simulink model "ASM_Traffic_V2X_Complete_Model_2"  (R2019a)
settings: Solver=ode1  StartTime=SIM.tstart.v  StopTime=Inf  FixedStep=SIM.StepSize.v  RelTol=1e-3
PostLoadFcn:
  | if any(exist('dsrtsu_mdlpostloadfcn', 'file') ~= 0), dsrtsu_mdlpostloadfcn('Execute', bdroot); end
  | try, asm_mdl_postloadfcn(bdroot, 'UpdateModel', 2200); catch, disp(lasterr); end,
undefined symbols (not defined in the file): _SensorPnts_1, _SensorPnts_13, _SensorPnts_17, _SensorPnts_21, _SensorPnts_25, _SensorPnts_29, _SensorPnts_33, _SensorPnts_37, _SensorPnts_41, _SensorPnts_45, _SensorPnts_49, _SensorPnts_5, _SensorPnts_53, _SensorPnts_57, _SensorPnts_9, _to_, CPT, G5A, ITS, MDL, rad, s_to_rpm, SIM
libraries: simulink x169, ASM_VehicleDynamics_lib x126, ASM_Traffic_lib x83, ASM_Utils_lib x49, mdbs x45, ASM_Environment_lib x17, dspindex x12, dsaV2xLibraryAux x10, dsmpblib x6, dsaV2xAsn1Library x4, dsaV2xLibrary x4, ASM_BrakeHydraulics_lib x4
(part 34 of 36)

== system ASM_Traffic_V2X_Complete_Model_2/MDL/Environment/Traffic/Sensors/Object_Sensor_3D/RadarEffects/Sensor1/RadarEffectsOutput/ResetPulse ==
  Enable[0|1] : Inport
  SensorActive[0|1] : Inport  Port=2
  Compare To Constant : simulink/Logic and Bit Operations/Compare To Constant  relop===  const=1  OutDataTypeStr=boolean
  Compare To Constant1 : simulink/Logic and Bit Operations/Compare To Constant  relop===  const=0  OutDataTypeStr=boolean
  Logical Operator1 : Logic  AllPortsSameDT=off  OutDataTypeStr=boolean
  Logical Operator2 : Logic  Operator=NAND  AllPortsSameDT=off  OutDataTypeStr=boolean
  Memory1 : Memory
  ResetPulse[0|1] : Outport
  wires:
  Memory1/1 -> Compare To Constant1/1
  Logical Operator2/1 -> Compare To Constant/1, Memory1/1
  SensorActive[0|1]/1 -> Logical Operator2/1
  Logical Operator1/1 -> ResetPulse[0|1]/1
  Compare To Constant/1 -> Logical Operator1/1
  Compare To Constant1/1 -> Logical Operator1/2
  Enable[0|1]/1 -> Logical Operator2/2

== system ASM_Traffic_V2X_Complete_Model_2/MDL/Environment/Traffic/Sensors/Object_Sensor_3D/RadarEffects/Sensor1/RadarEffectsOutput/SignalBus ==
  RadarEffect_Signals_In[] : Inport
  Bus Creator : BusCreator  Inputs=5
  Bus Selector1 : BusSelector  OutputSignals=ID[],Object_ID[],Dist_CoorSys_S[m],Angle_Hor_CoorSys_S[deg],Pos_ObjectPoint_CoorSys_E[x;y;z][m]
  RadarEffect_Signals_Out[] : Outport
  wires:
  RadarEffect_Signals_In[]/1 -> Bus Selector1/1
  Bus Creator/1 -> RadarEffect_Signals_Out[]/1
  Bus Selector1/4 -> Bus Creator/4  "<Angle_Hor_CoorSys_S[deg]>"
  Bus Selector1/5 -> Bus Creator/5  "<Pos_ObjectPoint_CoorSys_E[x;y;z][m]>"
  Bus Selector1/2 -> Bus Creator/2  "<Object_ID[]>"
  Bus Selector1/3 -> Bus Creator/3  "<Dist_CoorSys_S[m]>"
  Bus Selector1/1 -> Bus Creator/1  "<ID[]>"

== system ASM_Traffic_V2X_Complete_Model_2/MDL/Environment/Traffic/Sensors/Object_Sensor_3D/RadarEffects/Sensor2/RadarEffectsOutput/HoldSignals ==
  ResetPulse[0|1] : Inport
  RadarEffect_Signals_In[] : Inport  Port=2
  Enable : EnablePort
  Bus Selector1 : BusSelector  OutputSignals=ID[],Dist_CoorSys_S[m],v_CoorSys_S[m|s],Angle_Hor_CoorSys_S[deg],Angle_Ver_CoorSys_S[deg],RCS[dBm2],Object_ID[],Object_Type[],Pos_ObjectPoint_CoorSys_E[x;y;z][m],Pos_ObjectPoint_CoorSys_S[x;y;z][m]
  RADAR_SIGNALS_RESET_2 : ASM_Traffic_lib/Sensors/RadarEffects/RADAR_SIGNALS_RESET  ASMProperties=struct('Name','RADAR_SIGNALS_RESET','Version','1.0','Library','ASM_Traffic_lib')  ASMInstanceName=radar_signals_reset  ASMInstanceID=1
  RadarEffect_Signals_Out[] : Outport
  wires:
  ResetPulse[0|1]/1 -> RADAR_SIGNALS_RESET_2/1
  Bus Selector1/8 -> RADAR_SIGNALS_RESET_2/9  "<Object_Type[]>"
  Bus Selector1/3 -> RADAR_SIGNALS_RESET_2/4  "<v_CoorSys_S[m|s]>"
  Bus Selector1/7 -> RADAR_SIGNALS_RESET_2/8  "<Object_ID[]>"
  RadarEffect_Signals_In[]/1 -> Bus Selector1/1
  Bus Selector1/6 -> RADAR_SIGNALS_RESET_2/7  "<RCS[dBm2]>"
  Bus Selector1/5 -> RADAR_SIGNALS_RESET_2/6  "<Angle_Ver_CoorSys_S[deg]>"
  Bus Selector1/4 -> RADAR_SIGNALS_RESET_2/5  "<Angle_Hor_CoorSys_S[deg]>"
  Bus Selector1/2 -> RADAR_SIGNALS_RESET_2/3  "<Dist_CoorSys_S[m]>"
  Bus Selector1/10 -> RADAR_SIGNALS_RESET_2/11  "<Pos_ObjectPoint_CoorSys_S[x;y;z][m]>"
  Bus Selector1/1 -> RADAR_SIGNALS_RESET_2/2  "<ID[]>"
  Bus Selector1/9 -> RADAR_SIGNALS_RESET_2/10  "<Pos_ObjectPoint_CoorSys_E[x;y;z][m]>"
  RADAR_SIGNALS_RESET_2/1 -> RadarEffect_Signals_Out[]/1

== system ASM_Traffic_V2X_Complete_Model_2/MDL/Environment/Traffic/Sensors/Object_Sensor_3D/RadarEffects/Sensor2/RadarEffectsOutput/ResetPulse ==
  Enable[0|1] : Inport
  SensorActive[0|1] : Inport  Port=2
  Compare To Constant : simulink/Logic and Bit Operations/Compare To Constant  relop===  const=1  OutDataTypeStr=boolean
  Compare To Constant1 : simulink/Logic and Bit Operations/Compare To Constant  relop===  const=0  OutDataTypeStr=boolean
  Logical Operator1 : Logic  AllPortsSameDT=off  OutDataTypeStr=boolean
  Logical Operator2 : Logic  Operator=NAND  AllPortsSameDT=off  OutDataTypeStr=boolean
  Memory1 : Memory
  ResetPulse[0|1] : Outport
  wires:
  Memory1/1 -> Compare To Constant1/1
  Logical Operator2/1 -> Compare To Constant/1, Memory1/1
  SensorActive[0|1]/1 -> Logical Operator2/1
  Logical Operator1/1 -> ResetPulse[0|1]/1
  Compare To Constant/1 -> Logical Operator1/1
  Compare To Constant1/1 -> Logical Operator1/2
  Enable[0|1]/1 -> Logical Operator2/2

== system ASM_Traffic_V2X_Complete_Model_2/MDL/Environment/Traffic/Sensors/Object_Sensor_3D/RadarEffects/Sensor2/RadarEffectsOutput/SignalBus ==
  RadarEffect_Signals_In[] : Inport
  Bus Creator : BusCreator  Inputs=5
  Bus Selector1 : BusSelector  OutputSignals=ID[],Object_ID[],Dist_CoorSys_S[m],Angle_Hor_CoorSys_S[deg],Pos_ObjectPoint_CoorSys_E[x;y;z][m]
  RadarEffect_Signals_Out[] : Outport
  wires:
  RadarEffect_Signals_In[]/1 -> Bus Selector1/1
  Bus Creator/1 -> RadarEffect_Signals_Out[]/1
  Bus Selector1/4 -> Bus Creator/4  "<Angle_Hor_CoorSys_S[deg]>"
  Bus Selector1/5 -> Bus Creator/5  "<Pos_ObjectPoint_CoorSys_E[x;y;z][m]>"
  Bus Selector1/2 -> Bus Creator/2  "<Object_ID[]>"
  Bus Selector1/3 -> Bus Creator/3  "<Dist_CoorSys_S[m]>"
  Bus Selector1/1 -> Bus Creator/1  "<ID[]>"

== system ASM_Traffic_V2X_Complete_Model_2/MDL/Environment/Traffic/Sensors/Object_Sensor_3D/RadarEffects/Sensor3/RadarEffectsOutput/HoldSignals ==
  ResetPulse[0|1] : Inport
  RadarEffect_Signals_In[] : Inport  Port=2
  Enable : EnablePort
  Bus Selector1 : BusSelector  OutputSignals=ID[],Dist_CoorSys_S[m],v_CoorSys_S[m|s],Angle_Hor_CoorSys_S[deg],Angle_Ver_CoorSys_S[deg],RCS[dBm2],Object_ID[],Object_Type[],Pos_ObjectPoint_CoorSys_E[x;y;z][m],Pos_ObjectPoint_CoorSys_S[x;y;z][m]
  RADAR_SIGNALS_RESET_3 : ASM_Traffic_lib/Sensors/RadarEffects/RADAR_SIGNALS_RESET  ASMProperties=struct('Name','RADAR_SIGNALS_RESET','Version','1.0','Library','ASM_Traffic_lib')  ASMInstanceName=radar_signals_reset  ASMInstanceID=1
  RadarEffect_Signals_Out[] : Outport
  wires:
  RADAR_SIGNALS_RESET_3/1 -> RadarEffect_Signals_Out[]/1
  Bus Selector1/9 -> RADAR_SIGNALS_RESET_3/10  "<Pos_ObjectPoint_CoorSys_E[x;y;z][m]>"
  Bus Selector1/5 -> RADAR_SIGNALS_RESET_3/6  "<Angle_Ver_CoorSys_S[deg]>"
  Bus Selector1/4 -> RADAR_SIGNALS_RESET_3/5  "<Angle_Hor_CoorSys_S[deg]>"
  Bus Selector1/1 -> RADAR_SIGNALS_RESET_3/2  "<ID[]>"
  ResetPulse[0|1]/1 -> RADAR_SIGNALS_RESET_3/1
  Bus Selector1/6 -> RADAR_SIGNALS_RESET_3/7  "<RCS[dBm2]>"
  Bus Selector1/7 -> RADAR_SIGNALS_RESET_3/8  "<Object_ID[]>"
  Bus Selector1/3 -> RADAR_SIGNALS_RESET_3/4  "<v_CoorSys_S[m|s]>"
  RadarEffect_Signals_In[]/1 -> Bus Selector1/1
  Bus Selector1/10 -> RADAR_SIGNALS_RESET_3/11  "<Pos_ObjectPoint_CoorSys_S[x;y;z][m]>"
  Bus Selector1/8 -> RADAR_SIGNALS_RESET_3/9  "<Object_Type[]>"
  Bus Selector1/2 -> RADAR_SIGNALS_RESET_3/3  "<Dist_CoorSys_S[m]>"

== system ASM_Traffic_V2X_Complete_Model_2/MDL/Environment/Traffic/Sensors/Object_Sensor_3D/RadarEffects/Sensor3/RadarEffectsOutput/ResetPulse ==
  Enable[0|1] : Inport
  SensorActive[0|1] : Inport  Port=2
  Compare To Constant : simulink/Logic and Bit Operations/Compare To Constant  relop===  const=1  OutDataTypeStr=boolean
  Compare To Constant1 : simulink/Logic and Bit Operations/Compare To Constant  relop===  const=0  OutDataTypeStr=boolean
  Logical Operator1 : Logic  AllPortsSameDT=off  OutDataTypeStr=boolean
  Logical Operator2 : Logic  Operator=NAND  AllPortsSameDT=off  OutDataTypeStr=boolean
  Memory1 : Memory
  ResetPulse[0|1] : Outport
  wires:
  Memory1/1 -> Compare To Constant1/1
  Logical Operator2/1 -> Compare To Constant/1, Memory1/1
  SensorActive[0|1]/1 -> Logical Operator2/1
  Logical Operator1/1 -> ResetPulse[0|1]/1
  Compare To Constant/1 -> Logical Operator1/1
  Compare To Constant1/1 -> Logical Operator1/2
  Enable[0|1]/1 -> Logical Operator2/2

== system ASM_Traffic_V2X_Complete_Model_2/MDL/Environment/Traffic/Sensors/Object_Sensor_3D/RadarEffects/Sensor3/RadarEffectsOutput/SignalBus ==
  RadarEffect_Signals_In[] : Inport
  Bus Creator : BusCreator  Inputs=5
  Bus Selector1 : BusSelector  OutputSignals=ID[],Object_ID[],Dist_CoorSys_S[m],Angle_Hor_CoorSys_S[deg],Pos_ObjectPoint_CoorSys_E[x;y;z][m]
  RadarEffect_Signals_Out[] : Outport
  wires:
  RadarEffect_Signals_In[]/1 -> Bus Selector1/1
  Bus Creator/1 -> RadarEffect_Signals_Out[]/1
  Bus Selector1/4 -> Bus Creator/4  "<Angle_Hor_CoorSys_S[deg]>"
  Bus Selector1/5 -> Bus Creator/5  "<Pos_ObjectPoint_CoorSys_E[x;y;z][m]>"
  Bus Selector1/2 -> Bus Creator/2  "<Object_ID[]>"
  Bus Selector1/3 -> Bus Creator/3  "<Dist_CoorSys_S[m]>"
  Bus Selector1/1 -> Bus Creator/1  "<ID[]>"

== system ASM_Traffic_V2X_Complete_Model_2/MDLUserInterface/MotionDeskInterface/MOTION_DESK_INTERFACE/Traffic_Animation/Sensors_Animation/Sensor_Points/Object_Sensor_2D_Points/Calc_Object_Sensor_2D_Points/Sensor_Points ==
  Transform_In : Inport
  Angle_Hor_Rel[deg] : Inport  Port=2
  Distance[m] : Inport  Port=3
  Num_SensorRays_Used[] : Inport  Port=4
  Add : Sum
  CheckUnusedPoints : RelationalOperator  Operator=<  OutDataTypeStr=boolean  RndMeth=Nearest
  Concatenate : Concatenate  NumInputs=4  Mode=Multidimensional array
  Constant1 : Constant  Value=0.99999
  Cos : Trigonometry  Operator=cos
  Deg2Rad : Gain  Gain=pi/180
  Demux : Demux
  Demux1 : Demux
  Demux2 : Demux
  DownAway : Constant  Value=-999999
  ForIterator_Current : Subsystem  TreatAsAtomicUnit=on
  Product{,1..6} (7 alike) : Product
  Reshape : Reshape  OutputDimensionality=Row vector (2-D)
  Reshape1 : Reshape  OutputDimensionality=Row vector (2-D)
  Reshape2 : Reshape  OutputDimensionality=Row vector (2-D)
  Row0 : Selector  NumberOfDimensions=2  IndexMode=Zero-based  InputPortWidth=3  IndexOptions=Index vector (dialog),Index vector (dialog)  Indices=0,-1  OutputSizes=1,1
  Row1 : Selector  NumberOfDimensions=2  IndexMode=Zero-based  InputPortWidth=3  IndexOptions=Index vector (dialog),Index vector (dialog)  Indices=1,-1  OutputSizes=1,1
  Row2 : Selector  NumberOfDimensions=2  IndexMode=Zero-based  InputPortWidth=3  IndexOptions=Index vector (dialog),Index vector (dialog)  Indices=2,-1  OutputSizes=1,1
  Sin : Trigonometry
  Term : Terminator
  Term1 : Terminator
  Term2 : Terminator
  X : Sum  Inputs=+++
  Y : Sum  Inputs=+++
  Z : Sum  Inputs=+++
  dim_animation_point[] : Constant  Value=60
  init_animation_point[] : Constant  Value=zeros(1,60)  VectorParams1D=off
  x1 : Product
  y1 : Product
  y2 : Product
  y3 : Product
  Translate[x;y;z][m] : Outport
  wires:
  CheckUnusedPoints/1 -> Product/1
  Constant1/1 -> CheckUnusedPoints/2
  Product/1 -> Add/1
  DownAway/1 -> Product/2
  Add/1 -> Concatenate/3
  Reshape2/1 -> Add/2
  ForIterator_Current/3(flag_point_used[0|1]) -> CheckUnusedPoints/1, y3/1, y2/2
  Z/1 -> Reshape2/1
  Demux2/4 -> Z/3
  Product5/1 -> Z/2
  Product6/1 -> Z/1
  Demux2/3 -> Term2/1
  Demux2/2 -> Product5/1
  Demux2/1 -> Product6/1
  Row2/1 -> Demux2/1
  Y/1 -> Reshape1/1
  X/1 -> Reshape/1
  Concatenate/1 -> Translate[x;y;z][m]/1
  Demux1/4 -> Y/3
  Product3/1 -> Y/2
  Product4/1 -> Y/1
  Demux1/3 -> Term1/1
  Demux1/2 -> Product3/1
  Demux1/1 -> Product4/1
  Row1/1 -> Demux1/1
  Demux/4 -> X/3
  Product1/1 -> X/2
  Product2/1 -> X/1
  Demux/3 -> Term/1
  Demux/2 -> Product1/1
  Demux/1 -> Product2/1
  Row0/1 -> Demux/1
  y1/1 -> Product1/2, Product3/2
  x1/1 -> Product2/2, Product4/2, Product6/2, Product5/2
  Transform_In/1 -> Row0/1, Row1/1, Row2/1
  Sin/1 -> y1/2
  Cos/1 -> x1/2
  ForIterator_Current/1(distance_animation_point[m]) -> x1/1, y1/1
  Deg2Rad/1 -> Sin/1, Cos/1
  ForIterator_Current/2(angle_animation_point[deg]) -> Deg2Rad/1
  Num_SensorRays_Used[]/1 -> ForIterator_Current/3(num_sensor_rays[])
  dim_animation_point[]/1 -> ForIterator_Current/1(dim_animation_point[])
  Distance[m]/1 -> ForIterator_Current/4(distance_sensor_out)
  Angle_Hor_Rel[deg]/1 -> ForIterator_Current/5(angle_sensor_out)
  Reshape/1 -> y2/1
  Reshape1/1 -> y3/2
  init_animation_point[]/1 -> ForIterator_Current/2(init_animation_point[]), Concatenate/4
  y2/1 -> Concatenate/1
  y3/1 -> Concatenate/2

== system ASM_Traffic_V2X_Complete_Model_2/IO/I//O_Subsystem/Bus Configuration (1) - In/Simulated ECUs/DrivekitCAN/Drivekit/TX/PDUs/BRAKE_REPORT/PDU Features ==
  PDU Cyclic Timing Control : Subsystem
  _PDU Features_ : BusCreator  Inputs=1
  PDU Features : Outport
  wires:
  _PDU Features_/1 -> PDU Features/1  "PDU Features"
  PDU Cyclic Timing Control/1(PDU Cyclic Timing Control) -> _PDU Features_/1  "PDU Cyclic Timing Control"

== system ASM_Traffic_V2X_Complete_Model_2/IO/I//O_Subsystem/Bus Configuration (1) - In/Simulated ECUs/DrivekitCAN/Drivekit/TX/PDUs/BRAKE_REPORT/brake_dtcs ==
  ISignal Value : Subsystem
  _brake_dtcs_ : BusCreator  Inputs=1
  brake_dtcs : Outport
  wires:
  _brake_dtcs_/1 -> brake_dtcs/1  "brake_dtcs"
  ISignal Value/1(ISignal Value) -> _brake_dtcs_/1  "ISignal Value"

== system ASM_Traffic_V2X_Complete_Model_2/IO/I//O_Subsystem/Bus Configuration (1) - In/Simulated ECUs/DrivekitCAN/Drivekit/TX/PDUs/BRAKE_REPORT/brake_operator_override ==
  ISignal Value : Subsystem
  _brake_operator_override_ : BusCreator  Inputs=1
  brake_operator_override : Outport
  wires:
  _brake_operator_override_/1 -> brake_operator_override/1  "brake_operator_override"
  ISignal Value/1(ISignal Value) -> _brake_operator_override_/1  "ISignal Value"

== system ASM_Traffic_V2X_Complete_Model_2/IO/I//O_Subsystem/Bus Configuration (1) - In/Simulated ECUs/DrivekitCAN/Drivekit/TX/PDUs/BRAKE_REPORT/brake_report_enabled ==
  ISignal Value : Subsystem
  _brake_report_enabled_ : BusCreator  Inputs=1
  brake_report_enabled : Outport
  wires:
  _brake_report_enabled_/1 -> brake_report_enabled/1  "brake_report_enabled"
  ISignal Value/1(ISignal Value) -> _brake_report_enabled_/1  "ISignal Value"

== system ASM_Traffic_V2X_Complete_Model_2/IO/I//O_Subsystem/Bus Configuration (1) - In/Simulated ECUs/DrivekitCAN/Drivekit/TX/PDUs/BRAKE_REPORT/brake_report_magic ==
  ISignal Value : Subsystem
  _brake_report_magic_ : BusCreator  Inputs=1
  brake_report_magic : Outport
  wires:
  _brake_report_magic_/1 -> brake_report_magic/1  "brake_report_magic"
  ISignal Value/1(ISignal Value) -> _brake_report_magic_/1  "ISignal Value"

== system ASM_Traffic_V2X_Complete_Model_2/IO/I//O_Subsystem/Bus Configuration (1) - In/Simulated ECUs/DrivekitCAN/Drivekit/TX/PDUs/CHASSIS_CONTROL_REPORT/PDU Features ==
  PDU Cyclic Timing Control : Subsystem
  _PDU Features_ : BusCreator  Inputs=1
  PDU Features : Outport
  wires:
  _PDU Features_/1 -> PDU Features/1  "PDU Features"
  PDU Cyclic Timing Control/1(PDU Cyclic Timing Control) -> _PDU Features_/1  "PDU Cyclic Timing Control"

== system ASM_Traffic_V2X_Complete_Model_2/IO/I//O_Subsystem/Bus Configuration (1) - In/Simulated ECUs/DrivekitCAN/Drivekit/TX/PDUs/CHASSIS_CONTROL_REPORT/front_wipers ==
  ISignal Value : Subsystem
  _front_wipers_ : BusCreator  Inputs=1
  front_wipers : Outport
  wires:
  _front_wipers_/1 -> front_wipers/1  "front_wipers"
  ISignal Value/1(ISignal Value) -> _front_wipers_/1  "ISignal Value"

== system ASM_Traffic_V2X_Complete_Model_2/IO/I//O_Subsystem/Bus Configuration (1) - In/Simulated ECUs/DrivekitCAN/Drivekit/TX/PDUs/CHASSIS_CONTROL_REPORT/headlamps ==
  ISignal Value : Subsystem
  _headlamps_ : BusCreator  Inputs=1
  headlamps : Outport
  wires:
  _headlamps_/1 -> headlamps/1  "headlamps"
  ISignal Value/1(ISignal Value) -> _headlamps_/1  "ISignal Value"

== system ASM_Traffic_V2X_Complete_Model_2/IO/I//O_Subsystem/Bus Configuration (1) - In/Simulated ECUs/DrivekitCAN/Drivekit/TX/PDUs/CHASSIS_CONTROL_REPORT/horn ==
  ISignal Value : Subsystem
  _horn_ : BusCreator  Inputs=1
  horn : Outport
  wires:
  _horn_/1 -> horn/1  "horn"
  ISignal Value/1(ISignal Value) -> _horn_/1  "ISignal Value"

== system ASM_Traffic_V2X_Complete_Model_2/IO/I//O_Subsystem/Bus Configuration (1) - In/Simulated ECUs/DrivekitCAN/Drivekit/TX/PDUs/CHASSIS_CONTROL_REPORT/left_signal ==
  ISignal Value : Subsystem
  _left_signal_ : BusCreator  Inputs=1
  left_signal : Outport
  wires:
  _left_signal_/1 -> left_signal/1  "left_signal"
  ISignal Value/1(ISignal Value) -> _left_signal_/1  "ISignal Value"

== system ASM_Traffic_V2X_Complete_Model_2/IO/I//O_Subsystem/Bus Configuration (1) - In/Simulated ECUs/DrivekitCAN/Drivekit/TX/PDUs/CHASSIS_CONTROL_REPORT/rear_wiper ==
  ISignal Value : Subsystem
  _rear_wiper_ : BusCreator  Inputs=1
  rear_wiper : Outport
  wires:
  _rear_wiper_/1 -> rear_wiper/1  "rear_wiper"
  ISignal Value/1(ISignal Value) -> _rear_wiper_/1  "ISignal Value"

== system ASM_Traffic_V2X_Complete_Model_2/IO/I//O_Subsystem/Bus Configuration (1) - In/Simulated ECUs/DrivekitCAN/Drivekit/TX/PDUs/CHASSIS_CONTROL_REPORT/right_signal ==
  ISignal Value : Subsystem
  _right_signal_ : BusCreator  Inputs=1
  right_signal : Outport
  wires:
  _right_signal_/1 -> right_signal/1  "right_signal"
  ISignal Value/1(ISignal Value) -> _right_signal_/1  "ISignal Value"

== system ASM_Traffic_V2X_Complete_Model_2/IO/I//O_Subsystem/Bus Configuration (1) - In/Simulated ECUs/DrivekitCAN/Drivekit/TX/PDUs/CHASSIS_CONTROL_REPORT/vin_request ==
  ISignal Value : Subsystem
  _vin_request_ : BusCreator  Inputs=1
  vin_request : Outport
  wires:
  _vin_request_/1 -> vin_request/1  "vin_request"
  ISignal Value/1(ISignal Value) -> _vin_request_/1  "ISignal Value"

== system ASM_Traffic_V2X_Complete_Model_2/IO/I//O_Subsystem/Bus Configuration (1) - In/Simulated ECUs/DrivekitCAN/Drivekit/TX/PDUs/ESP12/CYL_PRES ==
  ISignal Value : Subsystem
  _CYL_PRES_ : BusCreator  Inputs=1
  CYL_PRES : Outport
  wires:
  _CYL_PRES_/1 -> CYL_PRES/1  "CYL_PRES"
  ISignal Value/1(ISignal Value) -> _CYL_PRES_/1  "ISignal Value"

== system ASM_Traffic_V2X_Complete_Model_2/IO/I//O_Subsystem/Bus Configuration (1) - In/Simulated ECUs/DrivekitCAN/Drivekit/TX/PDUs/ESP12/CYL_PRESS_DIAG ==
  ISignal Value : Subsystem
  _CYL_PRESS_DIAG_ : BusCreator  Inputs=1
  CYL_PRESS_DIAG : Outport
  wires:
  _CYL_PRESS_DIAG_/1 -> CYL_PRESS_DIAG/1  "CYL_PRESS_DIAG"
  ISignal Value/1(ISignal Value) -> _CYL_PRESS_DIAG_/1  "ISignal Value"

== system ASM_Traffic_V2X_Complete_Model_2/IO/I//O_Subsystem/Bus Configuration (1) - In/Simulated ECUs/DrivekitCAN/Drivekit/TX/PDUs/ESP12/CYL_PRES_STAT ==
  ISignal Value : Subsystem
  _CYL_PRES_STAT_ : BusCreator  Inputs=1
  CYL_PRES_STAT : Outport
  wires:
  _CYL_PRES_STAT_/1 -> CYL_PRES_STAT/1  "CYL_PRES_STAT"
  ISignal Value/1(ISignal Value) -> _CYL_PRES_STAT_/1  "ISignal Value"

== system ASM_Traffic_V2X_Complete_Model_2/IO/I//O_Subsystem/Bus Configuration (1) - In/Simulated ECUs/DrivekitCAN/Drivekit/TX/PDUs/ESP12/ESP12_AliveCounter ==
  ISignal Value : Subsystem
  _ESP12_AliveCounter_ : BusCreator  Inputs=1
  ESP12_AliveCounter : Outport
  wires:
  _ESP12_AliveCounter_/1 -> ESP12_AliveCounter/1  "ESP12_AliveCounter"
  ISignal Value/1(ISignal Value) -> _ESP12_AliveCounter_/1  "ISignal Value"

== system ASM_Traffic_V2X_Complete_Model_2/IO/I//O_Subsystem/Bus Configuration (1) - In/Simulated ECUs/DrivekitCAN/Drivekit/TX/PDUs/ESP12/ESP12_Checksum ==
  ISignal Value : Subsystem
  _ESP12_Checksum_ : BusCreator  Inputs=1
  ESP12_Checksum : Outport
  wires:
  _ESP12_Checksum_/1 -> ESP12_Checksum/1  "ESP12_Checksum"
  ISignal Value/1(ISignal Value) -> _ESP12_Checksum_/1  "ISignal Value"

== system ASM_Traffic_V2X_Complete_Model_2/IO/I//O_Subsystem/Bus Configuration (1) - In/Simulated ECUs/DrivekitCAN/Drivekit/TX/PDUs/ESP12/LAT_ACCEL ==
  ISignal Value : Subsystem
  _LAT_ACCEL_ : BusCreator  Inputs=1
  LAT_ACCEL : Outport
  wires:
  _LAT_ACCEL_/1 -> LAT_ACCEL/1  "LAT_ACCEL"
  ISignal Value/1(ISignal Value) -> _LAT_ACCEL_/1  "ISignal Value"

== system ASM_Traffic_V2X_Complete_Model_2/IO/I//O_Subsystem/Bus Configuration (1) - In/Simulated ECUs/DrivekitCAN/Drivekit/TX/PDUs/ESP12/LAT_ACCEL_DIAG ==
  ISignal Value : Subsystem
  _LAT_ACCEL_DIAG_ : BusCreator  Inputs=1
  LAT_ACCEL_DIAG : Outport
  wires:
  _LAT_ACCEL_DIAG_/1 -> LAT_ACCEL_DIAG/1  "LAT_ACCEL_DIAG"
  ISignal Value/1(ISignal Value) -> _LAT_ACCEL_DIAG_/1  "ISignal Value"

== system ASM_Traffic_V2X_Complete_Model_2/IO/I//O_Subsystem/Bus Configuration (1) - In/Simulated ECUs/DrivekitCAN/Drivekit/TX/PDUs/ESP12/LAT_ACCEL_STAT ==
  ISignal Value : Subsystem
  _LAT_ACCEL_STAT_ : BusCreator  Inputs=1
  LAT_ACCEL_STAT : Outport
  wires:
  _LAT_ACCEL_STAT_/1 -> LAT_ACCEL_STAT/1  "LAT_ACCEL_STAT"
  ISignal Value/1(ISignal Value) -> _LAT_ACCEL_STAT_/1  "ISignal Value"

== system ASM_Traffic_V2X_Complete_Model_2/IO/I//O_Subsystem/Bus Configuration (1) - In/Simulated ECUs/DrivekitCAN/Drivekit/TX/PDUs/ESP12/LONG_ACCEL ==
  ISignal Value : Subsystem
  _LONG_ACCEL_ : BusCreator  Inputs=1
  LONG_ACCEL : Outport
  wires:
  _LONG_ACCEL_/1 -> LONG_ACCEL/1  "LONG_ACCEL"
  ISignal Value/1(ISignal Value) -> _LONG_ACCEL_/1  "ISignal Value"

== system ASM_Traffic_V2X_Complete_Model_2/IO/I//O_Subsystem/Bus Configuration (1) - In/Simulated ECUs/DrivekitCAN/Drivekit/TX/PDUs/ESP12/LONG_ACCEL_DIAG ==
  ISignal Value : Subsystem
  _LONG_ACCEL_DIAG_ : BusCreator  Inputs=1
  LONG_ACCEL_DIAG : Outport
  wires:
  _LONG_ACCEL_DIAG_/1 -> LONG_ACCEL_DIAG/1  "LONG_ACCEL_DIAG"
  ISignal Value/1(ISignal Value) -> _LONG_ACCEL_DIAG_/1  "ISignal Value"

== system ASM_Traffic_V2X_Complete_Model_2/IO/I//O_Subsystem/Bus Configuration (1) - In/Simulated ECUs/DrivekitCAN/Drivekit/TX/PDUs/ESP12/LONG_ACCEL_STAT ==
  ISignal Value : Subsystem
  _LONG_ACCEL_STAT_ : BusCreator  Inputs=1
  LONG_ACCEL_STAT : Outport
  wires:
  _LONG_ACCEL_STAT_/1 -> LONG_ACCEL_STAT/1  "LONG_ACCEL_STAT"
  ISignal Value/1(ISignal Value) -> _LONG_ACCEL_STAT_/1  "ISignal Value"

== system ASM_Traffic_V2X_Complete_Model_2/IO/I//O_Subsystem/Bus Configuration (1) - In/Simulated ECUs/DrivekitCAN/Drivekit/TX/PDUs/ESP12/PDU Features ==
  PDU Cyclic Timing Control : Subsystem
  _PDU Features_ : BusCreator  Inputs=1
  PDU Features : Outport
  wires:
  _PDU Features_/1 -> PDU Features/1  "PDU Features"
  PDU Cyclic Timing Control/1(PDU Cyclic Timing Control) -> _PDU Features_/1  "PDU Cyclic Timing Control"

== system ASM_Traffic_V2X_Complete_Model_2/IO/I//O_Subsystem/Bus Configuration (1) - In/Simulated ECUs/DrivekitCAN/Drivekit/TX/PDUs/ESP12/YAW_RATE ==
  ISignal Value : Subsystem
  _YAW_RATE_ : BusCreator  Inputs=1
  YAW_RATE : Outport
  wires:
  _YAW_RATE_/1 -> YAW_RATE/1  "YAW_RATE"
  ISignal Value/1(ISignal Value) -> _YAW_RATE_/1  "ISignal Value"

== system ASM_Traffic_V2X_Complete_Model_2/IO/I//O_Subsystem/Bus Configuration (1) - In/Simulated ECUs/DrivekitCAN/Drivekit/TX/PDUs/ESP12/YAW_RATE_DIAG ==
  ISignal Value : Subsystem
  _YAW_RATE_DIAG_ : BusCreator  Inputs=1
  YAW_RATE_DIAG : Outport
  wires:
  _YAW_RATE_DIAG_/1 -> YAW_RATE_DIAG/1  "YAW_RATE_DIAG"
  ISignal Value/1(ISignal Value) -> _YAW_RATE_DIAG_/1  "ISignal Value"

== system ASM_Traffic_V2X_Complete_Model_2/IO/I//O_Subsystem/Bus Configuration (1) - In/Simulated ECUs/DrivekitCAN/Drivekit/TX/PDUs/ESP12/YAW_RATE_STAT ==
  ISignal Value : Subsystem
  _YAW_RATE_STAT_ : BusCreator  Inputs=1
  YAW_RATE_STAT : Outport
  wires:
  _YAW_RATE_STAT_/1 -> YAW_RATE_STAT/1  "YAW_RATE_STAT"
  ISignal Value/1(ISignal Value) -> _YAW_RATE_STAT_/1  "ISignal Value"

== system ASM_Traffic_V2X_Complete_Model_2/IO/I//O_Subsystem/Bus Configuration (1) - In/Simulated ECUs/DrivekitCAN/Drivekit/TX/PDUs/FAULT_REPORT/PDU Features ==
  PDU Cyclic Timing Control : Subsystem
  _PDU Features_ : BusCreator  Inputs=1
  PDU Features : Outport
  wires:
  _PDU Features_/1 -> PDU Features/1  "PDU Features"
  PDU Cyclic Timing Control/1(PDU Cyclic Timing Control) -> _PDU Features_/1  "PDU Cyclic Timing Control"

== system ASM_Traffic_V2X_Complete_Model_2/IO/I//O_Subsystem/Bus Configuration (1) - In/Simulated ECUs/DrivekitCAN/Drivekit/TX/PDUs/FAULT_REPORT/fault_dtcs ==
  ISignal Value : Subsystem
  _fault_dtcs_ : BusCreator  Inputs=1
  fault_dtcs : Outport
  wires:
  _fault_dtcs_/1 -> fault_dtcs/1  "fault_dtcs"
  ISignal Value/1(ISignal Value) -> _fault_dtcs_/1  "ISignal Value"

== system ASM_Traffic_V2X_Complete_Model_2/IO/I//O_Subsystem/Bus Configuration (1) - In/Simulated ECUs/DrivekitCAN/Drivekit/TX/PDUs/FAULT_REPORT/fault_origin_id ==
  ISignal Value : Subsystem
  _fault_origin_id_ : BusCreator  Inputs=1
  fault_origin_id : Outport
  wires:
  _fault_origin_id_/1 -> fault_origin_id/1  "fault_origin_id"
  ISignal Value/1(ISignal Value) -> _fault_origin_id_/1  "ISignal Value"

== system ASM_Traffic_V2X_Complete_Model_2/IO/I//O_Subsystem/Bus Configuration (1) - In/Simulated ECUs/DrivekitCAN/Drivekit/TX/PDUs/FAULT_REPORT/fault_report_magic ==
  ISignal Value : Subsystem
  _fault_report_magic_ : BusCreator  Inputs=1
  fault_report_magic : Outport
  wires:
  _fault_report_magic_/1 -> fault_report_magic/1  "fault_report_magic"
  ISignal Value/1(ISignal Value) -> _fault_report_magic_/1  "ISignal Value"

== system ASM_Traffic_V2X_Complete_Model_2/IO/I//O_Subsystem/Bus Configuration (1) - In/Simulated ECUs/DrivekitCAN/Drivekit/TX/PDUs/GPS_HEADING/Heading ==
  Input : Inport
  ISignal Value : Subsystem
  _Heading_ : BusCreator  Inputs=1
  Heading : Outport
  wires:
  _Heading_/1 -> Heading/1  "Heading"
  ISignal Value/1(ISignal Value) -> _Heading_/1  "ISignal Value"
  Input/1 -> ISignal Value/1(Input)

== system ASM_Traffic_V2X_Complete_Model_2/IO/I//O_Subsystem/Bus Configuration (1) - In/Simulated ECUs/DrivekitCAN/Drivekit/TX/PDUs/GPS_HEADING/PDU Features ==
  PDU Cyclic Timing Control : Subsystem
  _PDU Features_ : BusCreator  Inputs=1
  PDU Features : Outport
  wires:
  _PDU Features_/1 -> PDU Features/1  "PDU Features"
  PDU Cyclic Timing Control/1(PDU Cyclic Timing Control) -> _PDU Features_/1  "PDU Cyclic Timing Control"

== system ASM_Traffic_V2X_Complete_Model_2/IO/I//O_Subsystem/Bus Configuration (1) - In/Simulated ECUs/DrivekitCAN/Drivekit/TX/PDUs/GPS_LAT/Lat ==
  Input : Inport
  ISignal Value : Subsystem
  _Lat_ : BusCreator  Inputs=1
  Lat : Outport
  wires:
  _Lat_/1 -> Lat/1  "Lat"
  ISignal Value/1(ISignal Value) -> _Lat_/1  "ISignal Value"
  Input/1 -> ISignal Value/1(Input)

== system ASM_Traffic_V2X_Complete_Model_2/IO/I//O_Subsystem/Bus Configuration (1) - In/Simulated ECUs/DrivekitCAN/Drivekit/TX/PDUs/GPS_LAT/PDU Features ==
  PDU Cyclic Timing Control : Subsystem
  _PDU Features_ : BusCreator  Inputs=1
  PDU Features : Outport
  wires:
  _PDU Features_/1 -> PDU Features/1  "PDU Features"
  PDU Cyclic Timing Control/1(PDU Cyclic Timing Control) -> _PDU Features_/1  "PDU Cyclic Timing Control"

== system ASM_Traffic_V2X_Complete_Model_2/IO/I//O_Subsystem/Bus Configuration (1) - In/Simulated ECUs/DrivekitCAN/Drivekit/TX/PDUs/GPS_LONG/Long ==
  Input : Inport
  ISignal Value : Subsystem
  _Long_ : BusCreator  Inputs=1
  Long : Outport
  wires:
  _Long_/1 -> Long/1  "Long"
  ISignal Value/1(ISignal Value) -> _Long_/1  "ISignal Value"
  Input/1 -> ISignal Value/1(Input)

== system ASM_Traffic_V2X_Complete_Model_2/IO/I//O_Subsystem/Bus Configuration (1) - In/Simulated ECUs/DrivekitCAN/Drivekit/TX/PDUs/GPS_LONG/PDU Features ==
  PDU Cyclic Timing Control : Subsystem
  _PDU Features_ : BusCreator  Inputs=1
  PDU Features : Outport
  wires:
  _PDU Features_/1 -> PDU Features/1  "PDU Features"
  PDU Cyclic Timing Control/1(PDU Cyclic Timing Control) -> _PDU Features_/1  "PDU Cyclic Timing Control"

== system ASM_Traffic_V2X_Complete_Model_2/IO/I//O_Subsystem/Bus Configuration (1) - In/Simulated ECUs/DrivekitCAN/Drivekit/TX/PDUs/LANE_REPORT/PDU Features ==
  PDU Cyclic Timing Control : Subsystem
  _PDU Features_ : BusCreator  Inputs=1
  PDU Features : Outport
  wires:
  _PDU Features_/1 -> PDU Features/1  "PDU Features"
  PDU Cyclic Timing Control/1(PDU Cyclic Timing Control) -> _PDU Features_/1  "PDU Cyclic Timing Control"

== system ASM_Traffic_V2X_Complete_Model_2/IO/I//O_Subsystem/Bus Configuration (1) - In/Simulated ECUs/DrivekitCAN/Drivekit/TX/PDUs/LANE_REPORT/lane_number ==
  Input : Inport
  ISignal Value : Subsystem
  _lane_number_ : BusCreator  Inputs=1
  lane_number : Outport
  wires:
  _lane_number_/1 -> lane_number/1  "lane_number"
  ISignal Value/1(ISignal Value) -> _lane_number_/1  "ISignal Value"
  Input/1 -> ISignal Value/1(Input)

== system ASM_Traffic_V2X_Complete_Model_2/IO/I//O_Subsystem/Bus Configuration (1) - In/Simulated ECUs/DrivekitCAN/Drivekit/TX/PDUs/LANE_REPORT/left_marker_distance ==
  Input : Inport
  ISignal Value : Subsystem
  _left_marker_distance_ : BusCreator  Inputs=1
  left_marker_distance : Outport
  wires:
  _left_marker_distance_/1 -> left_marker_distance/1  "left_marker_distance"
  ISignal Value/1(ISignal Value) -> _left_marker_distance_/1  "ISignal Value"
  Input/1 -> ISignal Value/1(Input)

== system ASM_Traffic_V2X_Complete_Model_2/IO/I//O_Subsystem/Bus Configuration (1) - In/Simulated ECUs/DrivekitCAN/Drivekit/TX/PDUs/LANE_REPORT/right_marker_distance ==
  Input : Inport
  ISignal Value : Subsystem
  _right_marker_distance_ : BusCreator  Inputs=1
  right_marker_distance : Outport
  wires:
  _right_marker_distance_/1 -> right_marker_distance/1  "right_marker_distance"
  ISignal Value/1(ISignal Value) -> _right_marker_distance_/1  "ISignal Value"
  Input/1 -> ISignal Value/1(Input)

== system ASM_Traffic_V2X_Complete_Model_2/IO/I//O_Subsystem/Bus Configuration (1) - In/Simulated ECUs/DrivekitCAN/Drivekit/TX/PDUs/SAS11/PDU Features ==
  PDU Cyclic Timing Control : Subsystem
  _PDU Features_ : BusCreator  Inputs=1
  PDU Features : Outport
  wires:
  _PDU Features_/1 -> PDU Features/1  "PDU Features"
  PDU Cyclic Timing Control/1(PDU Cyclic Timing Control) -> _PDU Features_/1  "PDU Cyclic Timing Control"

== system ASM_Traffic_V2X_Complete_Model_2/IO/I//O_Subsystem/Bus Configuration (1) - In/Simulated ECUs/DrivekitCAN/Drivekit/TX/PDUs/SAS11/SAS_Angle ==
  Input : Inport
  ISignal Value : Subsystem
  _SAS_Angle_ : BusCreator  Inputs=1
  SAS_Angle : Outport
  wires:
  _SAS_Angle_/1 -> SAS_Angle/1  "SAS_Angle"
  ISignal Value/1(ISignal Value) -> _SAS_Angle_/1  "ISignal Value"
  Input/1 -> ISignal Value/1(Input)

== system ASM_Traffic_V2X_Complete_Model_2/IO/I//O_Subsystem/Bus Configuration (1) - In/Simulated ECUs/DrivekitCAN/Drivekit/TX/PDUs/SAS11/SAS_CheckSum ==
  ISignal Value : Subsystem
  _SAS_CheckSum_ : BusCreator  Inputs=1
  SAS_CheckSum : Outport
  wires:
  _SAS_CheckSum_/1 -> SAS_CheckSum/1  "SAS_CheckSum"
  ISignal Value/1(ISignal Value) -> _SAS_CheckSum_/1  "ISignal Value"

== system ASM_Traffic_V2X_Complete_Model_2/IO/I//O_Subsystem/Bus Configuration (1) - In/Simulated ECUs/DrivekitCAN/Drivekit/TX/PDUs/SAS11/SAS_MsgCount ==
  ISignal Value : Subsystem
  _SAS_MsgCount_ : BusCreator  Inputs=1
  SAS_MsgCount : Outport
  wires:
  _SAS_MsgCount_/1 -> SAS_MsgCount/1  "SAS_MsgCount"
  ISignal Value/1(ISignal Value) -> _SAS_MsgCount_/1  "ISignal Value"

== system ASM_Traffic_V2X_Complete_Model_2/IO/I//O_Subsystem/Bus Configuration (1) - In/Simulated ECUs/DrivekitCAN/Drivekit/TX/PDUs/SAS11/SAS_Speed ==
  ISignal Value : Subsystem
  _SAS_Speed_ : BusCreator  Inputs=1
  SAS_Speed : Outport
  wires:
  _SAS_Speed_/1 -> SAS_Speed/1  "SAS_Speed"
  ISignal Value/1(ISignal Value) -> _SAS_Speed_/1  "ISignal Value"

== system ASM_Traffic_V2X_Complete_Model_2/IO/I//O_Subsystem/Bus Configuration (1) - In/Simulated ECUs/DrivekitCAN/Drivekit/TX/PDUs/SAS11/SAS_Stat ==
  ISignal Value : Subsystem
  _SAS_Stat_ : BusCreator  Inputs=1
  SAS_Stat : Outport
  wires:
  _SAS_Stat_/1 -> SAS_Stat/1  "SAS_Stat"
  ISignal Value/1(ISignal Value) -> _SAS_Stat_/1  "ISignal Value"

== system ASM_Traffic_V2X_Complete_Model_2/IO/I//O_Subsystem/Bus Configuration (1) - In/Simulated ECUs/DrivekitCAN/Drivekit/TX/PDUs/STEERING_ANGLE_REPORT/PDU Features ==
  PDU Cyclic Timing Control : Subsystem
  _PDU Features_ : BusCreator  Inputs=1
  PDU Features : Outport
  wires:
  _PDU Features_/1 -> PDU Features/1  "PDU Features"
  PDU Cyclic Timing Control/1(PDU Cyclic Timing Control) -> _PDU Features_/1  "PDU Cyclic Timing Control"

== system ASM_Traffic_V2X_Complete_Model_2/IO/I//O_Subsystem/Bus Configuration (1) - In/Simulated ECUs/DrivekitCAN/Drivekit/TX/PDUs/STEERING_ANGLE_REPORT/steering_angle_report_errors ==
  ISignal Value : Subsystem
  _steering_angle_report_errors_ : BusCreator  Inputs=1
  steering_angle_report_errors : Outport
  wires:
  _steering_angle_report_errors_/1 -> steering_angle_report_errors/1  "steering_angle_report_errors"
  ISignal Value/1(ISignal Value) -> _steering_angle_report_errors_/1  "ISignal Value"

== system ASM_Traffic_V2X_Complete_Model_2/IO/I//O_Subsystem/Bus Configuration (1) - In/Simulated ECUs/DrivekitCAN/Drivekit/TX/PDUs/STEERING_ANGLE_REPORT/steering_angle_report_flags ==
  ISignal Value : Subsystem
  _steering_angle_report_flags_ : BusCreator  Inputs=1
  steering_angle_report_flags : Outport
  wires:
  _steering_angle_report_flags_/1 -> steering_angle_report_flags/1  "steering_angle_report_flags"
  ISignal Value/1(ISignal Value) -> _steering_angle_report_flags_/1  "ISignal Value"

== system ASM_Traffic_V2X_Complete_Model_2/IO/I//O_Subsystem/Bus Configuration (1) - In/Simulated ECUs/DrivekitCAN/Drivekit/TX/PDUs/STEERING_REPORT/PDU Features ==
  PDU Cyclic Timing Control : Subsystem
  _PDU Features_ : BusCreator  Inputs=1
  PDU Features : Outport
  wires:
  _PDU Features_/1 -> PDU Features/1  "PDU Features"
  PDU Cyclic Timing Control/1(PDU Cyclic Timing Control) -> _PDU Features_/1  "PDU Cyclic Timing Control"

== system ASM_Traffic_V2X_Complete_Model_2/IO/I//O_Subsystem/Bus Configuration (1) - In/Simulated ECUs/DrivekitCAN/Drivekit/TX/PDUs/STEERING_REPORT/steering_dtcs ==
  ISignal Value : Subsystem
  _steering_dtcs_ : BusCreator  Inputs=1
  steering_dtcs : Outport
  wires:
  _steering_dtcs_/1 -> steering_dtcs/1  "steering_dtcs"
  ISignal Value/1(ISignal Value) -> _steering_dtcs_/1  "ISignal Value"

== system ASM_Traffic_V2X_Complete_Model_2/IO/I//O_Subsystem/Bus Configuration (1) - In/Simulated ECUs/DrivekitCAN/Drivekit/TX/PDUs/STEERING_REPORT/steering_operator_override ==
  ISignal Value : Subsystem
  _steering_operator_override_ : BusCreator  Inputs=1
  steering_operator_override : Outport
  wires:
  _steering_operator_override_/1 -> steering_operator_override/1  "steering_operator_override"
  ISignal Value/1(ISignal Value) -> _steering_operator_override_/1  "ISignal Value"

== system ASM_Traffic_V2X_Complete_Model_2/IO/I//O_Subsystem/Bus Configuration (1) - In/Simulated ECUs/DrivekitCAN/Drivekit/TX/PDUs/STEERING_REPORT/steering_report_enabled ==
  ISignal Value : Subsystem
  _steering_report_enabled_ : BusCreator  Inputs=1
  steering_report_enabled : Outport
  wires:
  _steering_report_enabled_/1 -> steering_report_enabled/1  "steering_report_enabled"
  ISignal Value/1(ISignal Value) -> _steering_report_enabled_/1  "ISignal Value"

== system ASM_Traffic_V2X_Complete_Model_2/IO/I//O_Subsystem/Bus Configuration (1) - In/Simulated ECUs/DrivekitCAN/Drivekit/TX/PDUs/STEERING_REPORT/steering_report_magic ==
  ISignal Value : Subsystem
  _steering_report_magic_ : BusCreator  Inputs=1
  steering_report_magic : Outport
  wires:
  _steering_report_magic_/1 -> steering_report_magic/1  "steering_report_magic"
  ISignal Value/1(ISignal Value) -> _steering_report_magic_/1  "ISignal Value"

== system ASM_Traffic_V2X_Complete_Model_2/IO/I//O_Subsystem/Bus Configuration (1) - In/Simulated ECUs/DrivekitCAN/Drivekit/TX/PDUs/THROTTLE_REPORT/PDU Features ==
  PDU Cyclic Timing Control : Subsystem
  _PDU Features_ : BusCreator  Inputs=1
  PDU Features : Outport
  wires:
  _PDU Features_/1 -> PDU Features/1  "PDU Features"
  PDU Cyclic Timing Control/1(PDU Cyclic Timing Control) -> _PDU Features_/1  "PDU Cyclic Timing Control"

== system ASM_Traffic_V2X_Complete_Model_2/IO/I//O_Subsystem/Bus Configuration (1) - In/Simulated ECUs/DrivekitCAN/Drivekit/TX/PDUs/THROTTLE_REPORT/throttle_dtcs ==
  ISignal Value : Subsystem
  _throttle_dtcs_ : BusCreator  Inputs=1
  throttle_dtcs : Outport
  wires:
  _throttle_dtcs_/1 -> throttle_dtcs/1  "throttle_dtcs"
  ISignal Value/1(ISignal Value) -> _throttle_dtcs_/1  "ISignal Value"

== system ASM_Traffic_V2X_Complete_Model_2/IO/I//O_Subsystem/Bus Configuration (1) - In/Simulated ECUs/DrivekitCAN/Drivekit/TX/PDUs/THROTTLE_REPORT/throttle_operator_override ==
  ISignal Value : Subsystem
  _throttle_operator_override_ : BusCreator  Inputs=1
  throttle_operator_override : Outport
  wires:
  _throttle_operator_override_/1 -> throttle_operator_override/1  "throttle_operator_override"
  ISignal Value/1(ISignal Value) -> _throttle_operator_override_/1  "ISignal Value"

== system ASM_Traffic_V2X_Complete_Model_2/IO/I//O_Subsystem/Bus Configuration (1) - In/Simulated ECUs/DrivekitCAN/Drivekit/TX/PDUs/THROTTLE_REPORT/throttle_report_enabled ==
  ISignal Value : Subsystem
  _throttle_report_enabled_ : BusCreator  Inputs=1
  throttle_report_enabled : Outport
  wires:
  _throttle_report_enabled_/1 -> throttle_report_enabled/1  "throttle_report_enabled"
  ISignal Value/1(ISignal Value) -> _throttle_report_enabled_/1  "ISignal Value"

== system ASM_Traffic_V2X_Complete_Model_2/IO/I//O_Subsystem/Bus Configuration (1) - In/Simulated ECUs/DrivekitCAN/Drivekit/TX/PDUs/THROTTLE_REPORT/throttle_report_magic ==
  ISignal Value : Subsystem
  _throttle_report_magic_ : BusCreator  Inputs=1
  throttle_report_magic : Outport
  wires:
  _throttle_report_magic_/1 -> throttle_report_magic/1  "throttle_report_magic"
  ISignal Value/1(ISignal Value) -> _throttle_report_magic_/1  "ISignal Value"

== system ASM_Traffic_V2X_Complete_Model_2/IO/I//O_Subsystem/Bus Configuration (1) - In/Simulated ECUs/DrivekitCAN/Drivekit/TX/PDUs/WHL_SPD11/PDU Features ==
  PDU Cyclic Timing Control : Subsystem
  _PDU Features_ : BusCreator  Inputs=1
  PDU Features : Outport
  wires:
  _PDU Features_/1 -> PDU Features/1  "PDU Features"
  PDU Cyclic Timing Control/1(PDU Cyclic Timing Control) -> _PDU Features_/1  "PDU Cyclic Timing Control"

== system ASM_Traffic_V2X_Complete_Model_2/IO/I//O_Subsystem/Bus Configuration (1) - In/Simulated ECUs/DrivekitCAN/Drivekit/TX/PDUs/WHL_SPD11/WHL_SPD_AliveCounter_LSB ==
  ISignal Value : Subsystem
  _WHL_SPD_AliveCounter_LSB_ : BusCreator  Inputs=1
  WHL_SPD_AliveCounter_LSB : Outport
  wires:
  _WHL_SPD_AliveCounter_LSB_/1 -> WHL_SPD_AliveCounter_LSB/1  "WHL_SPD_AliveCounter_LSB"
  ISignal Value/1(ISignal Value) -> _WHL_SPD_AliveCounter_LSB_/1  "ISignal Value"

== system ASM_Traffic_V2X_Complete_Model_2/IO/I//O_Subsystem/Bus Configuration (1) - In/Simulated ECUs/DrivekitCAN/Drivekit/TX/PDUs/WHL_SPD11/WHL_SPD_AliveCounter_MSB ==
  ISignal Value : Subsystem
  _WHL_SPD_AliveCounter_MSB_ : BusCreator  Inputs=1
  WHL_SPD_AliveCounter_MSB : Outport
  wires:
  _WHL_SPD_AliveCounter_MSB_/1 -> WHL_SPD_AliveCounter_MSB/1  "WHL_SPD_AliveCounter_MSB"
  ISignal Value/1(ISignal Value) -> _WHL_SPD_AliveCounter_MSB_/1  "ISignal Value"

== system ASM_Traffic_V2X_Complete_Model_2/IO/I//O_Subsystem/Bus Configuration (1) - In/Simulated ECUs/DrivekitCAN/Drivekit/TX/PDUs/WHL_SPD11/WHL_SPD_Checksum_LSB ==
  ISignal Value : Subsystem
  _WHL_SPD_Checksum_LSB_ : BusCreator  Inputs=1
  WHL_SPD_Checksum_LSB : Outport
  wires:
  _WHL_SPD_Checksum_LSB_/1 -> WHL_SPD_Checksum_LSB/1  "WHL_SPD_Checksum_LSB"
  ISignal Value/1(ISignal Value) -> _WHL_SPD_Checksum_LSB_/1  "ISignal Value"

== system ASM_Traffic_V2X_Complete_Model_2/IO/I//O_Subsystem/Bus Configuration (1) - In/Simulated ECUs/DrivekitCAN/Drivekit/TX/PDUs/WHL_SPD11/WHL_SPD_Checksum_MSB ==
  ISignal Value : Subsystem
  _WHL_SPD_Checksum_MSB_ : BusCreator  Inputs=1
  WHL_SPD_Checksum_MSB : Outport
  wires:
  _WHL_SPD_Checksum_MSB_/1 -> WHL_SPD_Checksum_MSB/1  "WHL_SPD_Checksum_MSB"
  ISignal Value/1(ISignal Value) -> _WHL_SPD_Checksum_MSB_/1  "ISignal Value"

== system ASM_Traffic_V2X_Complete_Model_2/IO/I//O_Subsystem/Bus Configuration (1) - In/Simulated ECUs/DrivekitCAN/Drivekit/TX/PDUs/WHL_SPD11/WHL_SPD_FL ==
  Input : Inport
  ISignal Value : Subsystem
  _WHL_SPD_FL_ : BusCreator  Inputs=1
  WHL_SPD_FL : Outport
  wires:
  _WHL_SPD_FL_/1 -> WHL_SPD_FL/1  "WHL_SPD_FL"
  ISignal Value/1(ISignal Value) -> _WHL_SPD_FL_/1  "ISignal Value"
  Input/1 -> ISignal Value/1(Input)

== system ASM_Traffic_V2X_Complete_Model_2/IO/I//O_Subsystem/Bus Configuration (1) - In/Simulated ECUs/DrivekitCAN/Drivekit/TX/PDUs/WHL_SPD11/WHL_SPD_FR ==
  Input : Inport
  ISignal Value : Subsystem
  _WHL_SPD_FR_ : BusCreator  Inputs=1
  WHL_SPD_FR : Outport
  wires:
  _WHL_SPD_FR_/1 -> WHL_SPD_FR/1  "WHL_SPD_FR"
  ISignal Value/1(ISignal Value) -> _WHL_SPD_FR_/1  "ISignal Value"
  Input/1 -> ISignal Value/1(Input)

== system ASM_Traffic_V2X_Complete_Model_2/IO/I//O_Subsystem/Bus Configuration (1) - In/Simulated ECUs/DrivekitCAN/Drivekit/TX/PDUs/WHL_SPD11/WHL_SPD_RL ==
  Input : Inport
  ISignal Value : Subsystem
  _WHL_SPD_RL_ : BusCreator  Inputs=1
  WHL_SPD_RL : Outport
  wires:
  _WHL_SPD_RL_/1 -> WHL_SPD_RL/1  "WHL_SPD_RL"
  ISignal Value/1(ISignal Value) -> _WHL_SPD_RL_/1  "ISignal Value"
  Input/1 -> ISignal Value/1(Input)

== system ASM_Traffic_V2X_Complete_Model_2/IO/I//O_Subsystem/Bus Configuration (1) - In/Simulated ECUs/DrivekitCAN/Drivekit/TX/PDUs/WHL_SPD11/WHL_SPD_RR ==
  Input : Inport
  ISignal Value : Subsystem
  _WHL_SPD_RR_ : BusCreator  Inputs=1
  WHL_SPD_RR : Outport
  wires:
  _WHL_SPD_RR_/1 -> WHL_SPD_RR/1  "WHL_SPD_RR"
  ISignal Value/1(ISignal Value) -> _WHL_SPD_RR_/1  "ISignal Value"
  Input/1 -> ISignal Value/1(Input)

== system ASM_Traffic_V2X_Complete_Model_2/IO/I//O_Subsystem/Bus Configuration (1) - Out/Simulated ECUs/DrivekitCAN/Drivekit/RX/PDUs/BRAKE_COMMAND/brake_command_magic ==
  brake_command_magic : Inport
  ISignal Value : Subsystem
  _brake_command_magic_ : BusSelector  OutputSignals=ISignal Value
  wires:
  brake_command_magic/1 -> _brake_command_magic_/1  "brake_command_magic"
  _brake_command_magic_/1 -> ISignal Value/1(ISignal Value)  "<ISignal Value>"

== system ASM_Traffic_V2X_Complete_Model_2/IO/I//O_Subsystem/Bus Configuration (1) - Out/Simulated ECUs/DrivekitCAN/Drivekit/RX/PDUs/BRAKE_COMMAND/brake_pedal_command ==
  brake_pedal_command : Inport
  ISignal Value : Subsystem
  _brake_pedal_command_ : BusSelector  OutputSignals=ISignal Value
  wires:
  brake_pedal_command/1 -> _brake_pedal_command_/1  "brake_pedal_command"
  _brake_pedal_command_/1 -> ISignal Value/1(ISignal Value)  "<ISignal Value>"

== system ASM_Traffic_V2X_Complete_Model_2/IO/I//O_Subsystem/Bus Configuration (1) - Out/Simulated ECUs/DrivekitCAN/Drivekit/RX/PDUs/BRAKE_DISABLE/brake_disable_magic ==
  brake_disable_magic : Inport
  ISignal Value : Subsystem
  _brake_disable_magic_ : BusSelector  OutputSignals=ISignal Value
  wires:
  brake_disable_magic/1 -> _brake_disable_magic_/1  "brake_disable_magic"
  _brake_disable_magic_/1 -> ISignal Value/1(ISignal Value)  "<ISignal Value>"

== system ASM_Traffic_V2X_Complete_Model_2/IO/I//O_Subsystem/Bus Configuration (1) - Out/Simulated ECUs/DrivekitCAN/Drivekit/RX/PDUs/BRAKE_ENABLE/brake_enable_magic ==
  brake_enable_magic : Inport
  ISignal Value : Subsystem
  _brake_enable_magic_ : BusSelector  OutputSignals=ISignal Value
  wires:
  brake_enable_magic/1 -> _brake_enable_magic_/1  "brake_enable_magic"
  _brake_enable_magic_/1 -> ISignal Value/1(ISignal Value)  "<ISignal Value>"

== system ASM_Traffic_V2X_Complete_Model_2/IO/I//O_Subsystem/Bus Configuration (1) - Out/Simulated ECUs/DrivekitCAN/Drivekit/RX/PDUs/CHASSIS_CONTROL_COMMAND/front_wipers ==
  front_wipers : Inport
  ISignal Value : Subsystem
  _front_wipers_ : BusSelector  OutputSignals=ISignal Value
  wires:
  front_wipers/1 -> _front_wipers_/1  "front_wipers"
  _front_wipers_/1 -> ISignal Value/1(ISignal Value)  "<ISignal Value>"

== system ASM_Traffic_V2X_Complete_Model_2/IO/I//O_Subsystem/Bus Configuration (1) - Out/Simulated ECUs/DrivekitCAN/Drivekit/RX/PDUs/CHASSIS_CONTROL_COMMAND/headlamps ==
  headlamps : Inport
  ISignal Value : Subsystem
  _headlamps_ : BusSelector  OutputSignals=ISignal Value
  wires:
  headlamps/1 -> _headlamps_/1  "headlamps"
  _headlamps_/1 -> ISignal Value/1(ISignal Value)  "<ISignal Value>"

== system ASM_Traffic_V2X_Complete_Model_2/IO/I//O_Subsystem/Bus Configuration (1) - Out/Simulated ECUs/DrivekitCAN/Drivekit/RX/PDUs/CHASSIS_CONTROL_COMMAND/horn ==
  horn : Inport
  ISignal Value : Subsystem
  _horn_ : BusSelector  OutputSignals=ISignal Value
  wires:
  horn/1 -> _horn_/1  "horn"
  _horn_/1 -> ISignal Value/1(ISignal Value)  "<ISignal Value>"

== system ASM_Traffic_V2X_Complete_Model_2/IO/I//O_Subsystem/Bus Configuration (1) - Out/Simulated ECUs/DrivekitCAN/Drivekit/RX/PDUs/CHASSIS_CONTROL_COMMAND/left_signal ==
  left_signal : Inport
  ISignal Value : Subsystem
  _left_signal_ : BusSelector  OutputSignals=ISignal Value
  wires:
  left_signal/1 -> _left_signal_/1  "left_signal"
  _left_signal_/1 -> ISignal Value/1(ISignal Value)  "<ISignal Value>"

== system ASM_Traffic_V2X_Complete_Model_2/IO/I//O_Subsystem/Bus Configuration (1) - Out/Simulated ECUs/DrivekitCAN/Drivekit/RX/PDUs/CHASSIS_CONTROL_COMMAND/rear_wiper ==
  rear_wiper : Inport
  ISignal Value : Subsystem
  _rear_wiper_ : BusSelector  OutputSignals=ISignal Value
  wires:
  rear_wiper/1 -> _rear_wiper_/1  "rear_wiper"
  _rear_wiper_/1 -> ISignal Value/1(ISignal Value)  "<ISignal Value>"

== system ASM_Traffic_V2X_Complete_Model_2/IO/I//O_Subsystem/Bus Configuration (1) - Out/Simulated ECUs/DrivekitCAN/Drivekit/RX/PDUs/CHASSIS_CONTROL_COMMAND/right_signal ==
  right_signal : Inport
  ISignal Value : Subsystem
  _right_signal_ : BusSelector  OutputSignals=ISignal Value
  wires:
  right_signal/1 -> _right_signal_/1  "right_signal"
  _right_signal_/1 -> ISignal Value/1(ISignal Value)  "<ISignal Value>"

== system ASM_Traffic_V2X_Complete_Model_2/IO/I//O_Subsystem/Bus Configuration (1) - Out/Simulated ECUs/DrivekitCAN/Drivekit/RX/PDUs/CHASSIS_CONTROL_COMMAND/vin ==
  vin : Inport
  ISignal Value : Subsystem
  _vin_ : BusSelector  OutputSignals=ISignal Value
  wires:
  vin/1 -> _vin_/1  "vin"
  _vin_/1 -> ISignal Value/1(ISignal Value)  "<ISignal Value>"

== system ASM_Traffic_V2X_Complete_Model_2/IO/I//O_Subsystem/Bus Configuration (1) - Out/Simulated ECUs/DrivekitCAN/Drivekit/RX/PDUs/STEERING_ANGLE_COMMAND/steering_angle_cmd_angle ==
  steering_angle_cmd_angle : Inport
  ISignal Value : Subsystem
  _steering_angle_cmd_angle_ : BusSelector  OutputSignals=ISignal Value
  wires:
  steering_angle_cmd_angle/1 -> _steering_angle_cmd_angle_/1  "steering_angle_cmd_angle"
  _steering_angle_cmd_angle_/1 -> ISignal Value/1(ISignal Value)  "<ISignal Value>"

== system ASM_Traffic_V2X_Complete_Model_2/IO/I//O_Subsystem/Bus Configuration (1) - Out/Simulated ECUs/DrivekitCAN/Drivekit/RX/PDUs/STEERING_ANGLE_COMMAND/steering_angle_cmd_flags ==
  steering_angle_cmd_flags : Inport
  ISignal Value : Subsystem
  _steering_angle_cmd_flags_ : BusSelector  OutputSignals=ISignal Value
  wires:
  steering_angle_cmd_flags/1 -> _steering_angle_cmd_flags_/1  "steering_angle_cmd_flags"
  _steering_angle_cmd_flags_/1 -> ISignal Value/1(ISignal Value)  "<ISignal Value>"

== system ASM_Traffic_V2X_Complete_Model_2/IO/I//O_Subsystem/Bus Configuration (1) - Out/Simulated ECUs/DrivekitCAN/Drivekit/RX/PDUs/STEERING_ANGLE_COMMAND/steering_angle_cmd_max_velocity ==
  steering_angle_cmd_max_velocity : Inport
  ISignal Value : Subsystem
  _steering_angle_cmd_max_velocity_ : BusSelector  OutputSignals=ISignal Value
  wires:
  steering_angle_cmd_max_velocity/1 -> _steering_angle_cmd_max_velocity_/1  "steering_angle_cmd_max_velocity"
  _steering_angle_cmd_max_velocity_/1 -> ISignal Value/1(ISignal Value)  "<ISignal Value>"

== system ASM_Traffic_V2X_Complete_Model_2/IO/I//O_Subsystem/Bus Configuration (1) - Out/Simulated ECUs/DrivekitCAN/Drivekit/RX/PDUs/STEERING_DISABLE/steering_disable_magic ==
  steering_disable_magic : Inport
  ISignal Value : Subsystem
  _steering_disable_magic_ : BusSelector  OutputSignals=ISignal Value
  wires:
  steering_disable_magic/1 -> _steering_disable_magic_/1  "steering_disable_magic"
  _steering_disable_magic_/1 -> ISignal Value/1(ISignal Value)  "<ISignal Value>"

== system ASM_Traffic_V2X_Complete_Model_2/IO/I//O_Subsystem/Bus Configuration (1) - Out/Simulated ECUs/DrivekitCAN/Drivekit/RX/PDUs/STEERING_ENABLE/steering_enable_magic ==
  steering_enable_magic : Inport
  ISignal Value : Subsystem
  _steering_enable_magic_ : BusSelector  OutputSignals=ISignal Value
  wires:
  steering_enable_magic/1 -> _steering_enable_magic_/1  "steering_enable_magic"
  _steering_enable_magic_/1 -> ISignal Value/1(ISignal Value)  "<ISignal Value>"

== system ASM_Traffic_V2X_Complete_Model_2/IO/I//O_Subsystem/Bus Configuration (1) - Out/Simulated ECUs/DrivekitCAN/Drivekit/RX/PDUs/STEERING_TORQUE_COMMAND/steering_command_magic ==
  steering_command_magic : Inport
  ISignal Value : Subsystem
  _steering_command_magic_ : BusSelector  OutputSignals=ISignal Value
  wires:
  steering_command_magic/1 -> _steering_command_magic_/1  "steering_command_magic"
  _steering_command_magic_/1 -> ISignal Value/1(ISignal Value)  "<ISignal Value>"
